simulink model "fil_videosharp_sim"  (R2018b)
settings: Solver=FixedStepDiscrete  StartTime=0.0  StopTime=inf  RelTol=1e-3
InitFcn:
  | filter = fi(fspecial('unsharp'),1,16,12);
  | 
  | % video size excluding the blanking periods
  | fileName = get_param('fil_videosharp_sim/From Multimedia File',  'inputFilename');
  | x=mmfileinfo(fileName);
  | v = x.Video ;
  | H = v.Height;
  | W = v.Width;
  | %H = 176;
  | %W = 240;
  | activeVideoSize = [H W];
  | 
  | % horizontal and vertical blanking
  | hBlanking = 0;
  | vBlanking = 0;
undefined symbols (not defined in the file): gcbh, gray, none, NumBits1, NumBits2, Rec, SDTV, Slope1, Slope2, videoinput
libraries: simulink x19, visionconversions x3, dspsigattribs x3, visiongeotforms x3, dspbuff3 x3, hdlsllib x3, visionsinks x1, dspvision x1, imaqlib x1, simulink_need_slupdate x1, fillib x1
(part 2 of 3)

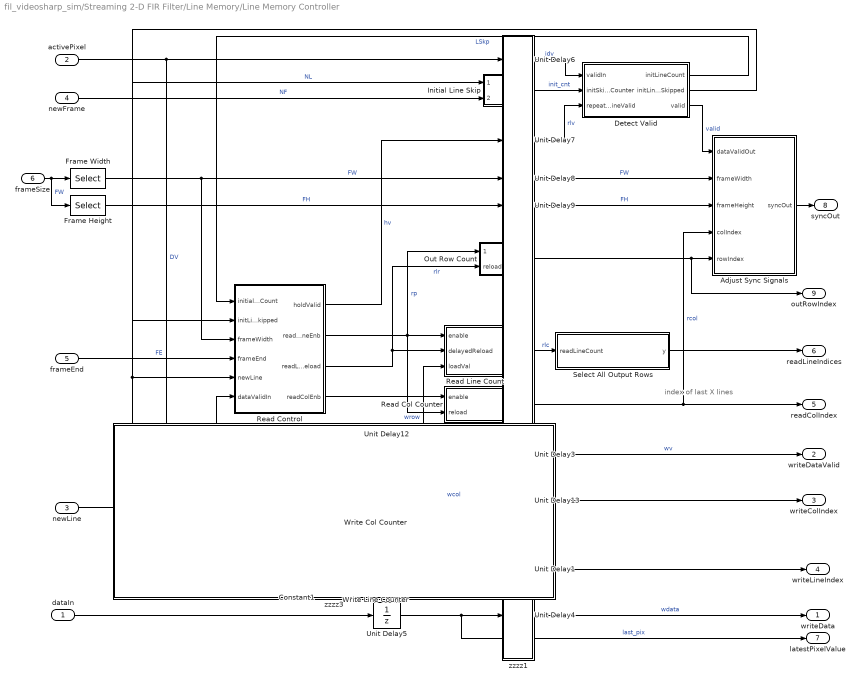
== system fil_videosharp_sim/Streaming 2-D FIR Filter/Line Memory/Line Memory Controller ==
  note: index of last X lines
  dataIn : Inport
  activePixel : Inport  Port=2
  newLine : Inport  Port=3
  newFrame : Inport  Port=4
  frameEnd : Inport  Port=5
  frameSize : Inport  Port=6
  Adjust Sync Signals : Subsystem
  Constant1 : Constant  Value=0  OutDataTypeStr=boolean
  Detect Valid : Subsystem
  Frame Height : Selector  InputPortWidth=2  IndexOptions=Index vector (dialog)  Indices=[1]  OutputSizes=1
  Frame Width : Selector  InputPortWidth=2  IndexOptions=Index vector (dialog)  Indices=[2]  OutputSizes=1
  Initial Line Skip : Subsystem  mask{INIT_VAL=0, STEP_VAL=1, MIN_VAL=0, MAX_VAL=floor(nL/2)+1, RELOADTYPE=Specified reload value, RELOAD_VAL=1, STOPTYPE=stop at specified count, STOP_VAL=floor(nL/2)+1, ROLLTYPE=roll-over to initial value, ROLL_VAL=2, SIGN=unsigned, WLTYPE=auto, WL=10}
      mask prompts: INIT_VAL "Initial value"; STEP_VAL "Step value"; MIN_VAL "Minimum value"; MAX_VAL "Maximum value"; RELOADTYPE "reload to:"; RELOAD_VAL "reload value"; STOPTYPE "Stop at:"; STOP_VAL "Stop at / Roll over from:"; ROLLTYPE "Roll over to:"; ROLL_VAL "Roll-over value"; SIGN "output data is :"; WLTYPE "World length option:"; WL "Word length"
      mask TypeOptions RELOADTYPE: Initial value | Specified reload value
      mask Callback RELOADTYPE:
      | maskStr = get_param(gcb,'MaskValues');
      | maskvisi = get_param(gcb,'MaskVisibilities');
      | maskenebles = get_param(gcb,'MaskEnables');
      | 
      | if strcmp(maskStr{5},'Specified reload value')
      |     maskenebles{6,1}='on';
      |     maskvisi{6,1}='on';
      | else
      |     maskenebles{6,1}='off';
      |     maskvisi{6,1}='off';
      | end
      | 
      | set_param(gcb,'MaskValues',maskStr);
      | set_param(gcb,'MaskVisibilities',maskvisi);
      | set_param(gcb,'MaskEnables',maskenebles);
      mask TypeOptions STOPTYPE: do not stop - auto roll-over | stop at specified count
      mask Callback STOPTYPE:
      | maskStr = get_param(gcb,'MaskValues');
      | maskvisi = get_param(gcb,'MaskVisibilities');
      | maskenebles = get_param(gcb,'MaskEnables');
      | 
      | if strcmp(maskStr{7},'do not stop - auto roll-over')
      |     maskenebles{9,1}='on';
      |     maskvisi{9,1}='on';
      | 
      |     if strcmp(maskStr{9},'roll-over to specified value')
      |         maskenebles{10,1}='on';
      |         maskvisi{10,1}='on';
      |     else
      |         maskenebles{10,1}='off';
      |         maskvisi{10,1}='off';
      | 
      |     end
      | else
      |     maskenebles{9,1}='off';
      |     maskvisi{9,1}='off';
      |     maskenebles{10,1}='off';
      |     maskvisi{10,1}='off';
      | end
      | set_param(gcb,'MaskValues',maskStr);
      | set_param(gcb,'MaskVisibilities',maskvisi);
      | set_param(gcb,'MaskEnables',maskenebles);
      mask TypeOptions ROLLTYPE: roll-over to initial value | roll-over to specified value
      mask Callback ROLLTYPE:
      | maskStr = get_param(gcb,'MaskValues');
      | maskvisi = get_param(gcb,'MaskVisibilities');
      | maskenebles = get_param(gcb,'MaskEnables');
      | 
      | if strcmp(maskStr{9},'roll-over to specified value') ...
      |         && strcmp(maskStr{7},'do not stop - auto roll-over')
      |     maskenebles{10,1}='on';
      |     maskvisi{10,1}='on';
      | else
      |     maskenebles{10,1}='off';
      |     maskvisi{10,1}='off';
      | end
      | 
      | set_param(gcb,'MaskValues',maskStr);
      | set_param(gcb,'MaskVisibilities',maskvisi);
      | set_param(gcb,'MaskEnables',maskenebles);
      mask TypeOptions SIGN: signed | unsigned
      mask TypeOptions WLTYPE: auto | specified
      mask Callback WLTYPE:
      | maskStr = get_param(gcb,'MaskValues');
      | maskvisi = get_param(gcb,'MaskVisibilities');
      | maskenebles = get_param(gcb,'MaskEnables');
      | 
      | if strcmp(maskStr{12},'specified')
      |     maskenebles{13,1}='on';
      |     maskvisi{13,1}='on';
      | else
      |     maskenebles{13,1}='off';
      |     maskvisi{13,1}='off';
      | end
      | 
      | set_param(gcb,'MaskValues',maskStr);
      | set_param(gcb,'MaskVisibilities',maskvisi);
      | set_param(gcb,'MaskEnables',maskenebles);
  Out Row Count : Subsystem  mask{INIT_VAL=0, STEP_VAL=1, MIN_VAL=0, MAX_VAL=maxnr, RELOADTYPE=Initial value, RELOAD_VAL=1, STOPTYPE=stop at specified count, STOP_VAL=maxnr, ROLLTYPE=roll-over to initial value, ROLL_VAL=2, SIGN=unsigned, WLTYPE=auto, WL=10}
      mask prompts: INIT_VAL "Initial value"; STEP_VAL "Step value"; MIN_VAL "Minimum value"; MAX_VAL "Maximum value"; RELOADTYPE "reload to:"; RELOAD_VAL "reload value"; STOPTYPE "Stop at:"; STOP_VAL "Stop at / Roll over from:"; ROLLTYPE "Roll over to:"; ROLL_VAL "Roll-over value"; SIGN "output data is :"; WLTYPE "World length option:"; WL "Word length"
      mask TypeOptions RELOADTYPE: Initial value | Specified reload value
      mask Callback RELOADTYPE:
      | maskStr = get_param(gcb,'MaskValues');
      | maskvisi = get_param(gcb,'MaskVisibilities');
      | maskenebles = get_param(gcb,'MaskEnables');
      | 
      | if strcmp(maskStr{5},'Specified reload value')
      |     maskenebles{6,1}='on';
      |     maskvisi{6,1}='on';
      | else
      |     maskenebles{6,1}='off';
      |     maskvisi{6,1}='off';
      | end
      | 
      | set_param(gcb,'MaskValues',maskStr);
      | set_param(gcb,'MaskVisibilities',maskvisi);
      | set_param(gcb,'MaskEnables',maskenebles);
      mask TypeOptions STOPTYPE: do not stop - auto roll-over | stop at specified count
      mask Callback STOPTYPE:
      | maskStr = get_param(gcb,'MaskValues');
      | maskvisi = get_param(gcb,'MaskVisibilities');
      | maskenebles = get_param(gcb,'MaskEnables');
      | 
      | if strcmp(maskStr{7},'do not stop - auto roll-over')
      |     maskenebles{9,1}='on';
      |     maskvisi{9,1}='on';
      | 
      |     if strcmp(maskStr{9},'roll-over to specified value')
      |         maskenebles{10,1}='on';
      |         maskvisi{10,1}='on';
      |     else
      |         maskenebles{10,1}='off';
      |         maskvisi{10,1}='off';
      | 
      |     end
      | else
      |     maskenebles{9,1}='off';
      |     maskvisi{9,1}='off';
      |     maskenebles{10,1}='off';
      |     maskvisi{10,1}='off';
      | end
      | set_param(gcb,'MaskValues',maskStr);
      | set_param(gcb,'MaskVisibilities',maskvisi);
      | set_param(gcb,'MaskEnables',maskenebles);
      mask TypeOptions ROLLTYPE: roll-over to initial value | roll-over to specified value
      mask Callback ROLLTYPE:
      | maskStr = get_param(gcb,'MaskValues');
      | maskvisi = get_param(gcb,'MaskVisibilities');
      | maskenebles = get_param(gcb,'MaskEnables');
      | 
      | if strcmp(maskStr{9},'roll-over to specified value') ...
      |         && strcmp(maskStr{7},'do not stop - auto roll-over')
      |     maskenebles{10,1}='on';
      |     maskvisi{10,1}='on';
      | else
      |     maskenebles{10,1}='off';
      |     maskvisi{10,1}='off';
      | end
      | 
      | set_param(gcb,'MaskValues',maskStr);
      | set_param(gcb,'MaskVisibilities',maskvisi);
      | set_param(gcb,'MaskEnables',maskenebles);
      mask TypeOptions SIGN: signed | unsigned
      mask TypeOptions WLTYPE: auto | specified
      mask Callback WLTYPE:
      | maskStr = get_param(gcb,'MaskValues');
      | maskvisi = get_param(gcb,'MaskVisibilities');
      | maskenebles = get_param(gcb,'MaskEnables');
      | 
      | if strcmp(maskStr{12},'specified')
      |     maskenebles{13,1}='on';
      |     maskvisi{13,1}='on';
      | else
      |     maskenebles{13,1}='off';
      |     maskvisi{13,1}='off';
      | end
      | 
      | set_param(gcb,'MaskValues',maskStr);
      | set_param(gcb,'MaskVisibilities',maskvisi);
      | set_param(gcb,'MaskEnables',maskenebles);
  Read Col Counter : Subsystem  mask{INIT_VAL=0, STEP_VAL=1, MIN_VAL=0, MAX_VAL=maxnc-1, RELOADTYPE=Initial value, RELOAD_VAL=3, STOPTYPE=stop at specified count, STOP_VAL=maxnc-1, ROLLTYPE=roll-over to specified value, ROLL_VAL=2, SIGN=unsigned, WLTYPE=auto, WL=10}
      mask prompts: INIT_VAL "Initial value"; STEP_VAL "Step value"; MIN_VAL "Minimum value"; MAX_VAL "Maximum value"; RELOADTYPE "reload to:"; RELOAD_VAL "reload value"; STOPTYPE "Stop at:"; STOP_VAL "Stop at / Roll over from:"; ROLLTYPE "Roll over to:"; ROLL_VAL "Roll-over value"; SIGN "output data is :"; WLTYPE "World length option:"; WL "Word length"
      mask TypeOptions RELOADTYPE: Initial value | Specified reload value
      mask Callback RELOADTYPE:
      | maskStr = get_param(gcb,'MaskValues');
      | maskvisi = get_param(gcb,'MaskVisibilities');
      | maskenebles = get_param(gcb,'MaskEnables');
      | 
      | if strcmp(maskStr{5},'Specified reload value')
      |     maskenebles{6,1}='on';
      |     maskvisi{6,1}='on';
      | else
      |     maskenebles{6,1}='off';
      |     maskvisi{6,1}='off';
      | end
      | 
      | set_param(gcb,'MaskValues',maskStr);
      | set_param(gcb,'MaskVisibilities',maskvisi);
      | set_param(gcb,'MaskEnables',maskenebles);
      mask TypeOptions STOPTYPE: do not stop - auto roll-over | stop at specified count
      mask Callback STOPTYPE:
      | maskStr = get_param(gcb,'MaskValues');
      | maskvisi = get_param(gcb,'MaskVisibilities');
      | maskenebles = get_param(gcb,'MaskEnables');
      | 
      | if strcmp(maskStr{7},'do not stop - auto roll-over')
      |     maskenebles{9,1}='on';
      |     maskvisi{9,1}='on';
      | 
      |     if strcmp(maskStr{9},'roll-over to specified value')
      |         maskenebles{10,1}='on';
      |         maskvisi{10,1}='on';
      |     else
      |         maskenebles{10,1}='off';
      |         maskvisi{10,1}='off';
      | 
      |     end
      | else
      |     maskenebles{9,1}='off';
      |     maskvisi{9,1}='off';
      |     maskenebles{10,1}='off';
      |     maskvisi{10,1}='off';
      | end
      | set_param(gcb,'MaskValues',maskStr);
      | set_param(gcb,'MaskVisibilities',maskvisi);
      | set_param(gcb,'MaskEnables',maskenebles);
      mask TypeOptions ROLLTYPE: roll-over to initial value | roll-over to specified value
      mask Callback ROLLTYPE:
      | maskStr = get_param(gcb,'MaskValues');
      | maskvisi = get_param(gcb,'MaskVisibilities');
      | maskenebles = get_param(gcb,'MaskEnables');
      | 
      | if strcmp(maskStr{9},'roll-over to specified value') ...
      |         && strcmp(maskStr{7},'do not stop - auto roll-over')
      |     maskenebles{10,1}='on';
      |     maskvisi{10,1}='on';
      | else
      |     maskenebles{10,1}='off';
      |     maskvisi{10,1}='off';
      | end
      | 
      | set_param(gcb,'MaskValues',maskStr);
      | set_param(gcb,'MaskVisibilities',maskvisi);
      | set_param(gcb,'MaskEnables',maskenebles);
      mask TypeOptions SIGN: signed | unsigned
      mask TypeOptions WLTYPE: auto | specified
      mask Callback WLTYPE:
      | maskStr = get_param(gcb,'MaskValues');
      | maskvisi = get_param(gcb,'MaskVisibilities');
      | maskenebles = get_param(gcb,'MaskEnables');
      | 
      | if strcmp(maskStr{12},'specified')
      |     maskenebles{13,1}='on';
      |     maskvisi{13,1}='on';
      | else
      |     maskenebles{13,1}='off';
      |     maskvisi{13,1}='off';
      | end
      | 
      | set_param(gcb,'MaskValues',maskStr);
      | set_param(gcb,'MaskVisibilities',maskvisi);
      | set_param(gcb,'MaskEnables',maskenebles);
  Read Control : Subsystem
  Read Line Count : Subsystem
  Select All Output Rows : MATLAB Function  TreatAsAtomicUnit=on
  Unit Delay{1,3..9,12..13} (10 alike) : UnitDelay  SampleTime=-1
  Write Col Counter : Subsystem  mask{INIT_VAL=0, STEP_VAL=1, MIN_VAL=0, MAX_VAL=maxnc-1, RELOADTYPE=Initial value, RELOAD_VAL=3, STOPTYPE=stop at specified count, STOP_VAL=maxnc-1, ROLLTYPE=roll-over to specified value, ROLL_VAL=2, SIGN=unsigned, WLTYPE=auto, WL=10}
      mask prompts: INIT_VAL "Initial value"; STEP_VAL "Step value"; MIN_VAL "Minimum value"; MAX_VAL "Maximum value"; RELOADTYPE "reload to:"; RELOAD_VAL "reload value"; STOPTYPE "Stop at:"; STOP_VAL "Stop at / Roll over from:"; ROLLTYPE "Roll over to:"; ROLL_VAL "Roll-over value"; SIGN "output data is :"; WLTYPE "World length option:"; WL "Word length"
      mask TypeOptions RELOADTYPE: Initial value | Specified reload value
      mask Callback RELOADTYPE:
      | maskStr = get_param(gcb,'MaskValues');
      | maskvisi = get_param(gcb,'MaskVisibilities');
      | maskenebles = get_param(gcb,'MaskEnables');
      | 
      | if strcmp(maskStr{5},'Specified reload value')
      |     maskenebles{6,1}='on';
      |     maskvisi{6,1}='on';
      | else
      |     maskenebles{6,1}='off';
      |     maskvisi{6,1}='off';
      | end
      | 
      | set_param(gcb,'MaskValues',maskStr);
      | set_param(gcb,'MaskVisibilities',maskvisi);
      | set_param(gcb,'MaskEnables',maskenebles);
      mask TypeOptions STOPTYPE: do not stop - auto roll-over | stop at specified count
      mask Callback STOPTYPE:
      | maskStr = get_param(gcb,'MaskValues');
      | maskvisi = get_param(gcb,'MaskVisibilities');
      | maskenebles = get_param(gcb,'MaskEnables');
      | 
      | if strcmp(maskStr{7},'do not stop - auto roll-over')
      |     maskenebles{9,1}='on';
      |     maskvisi{9,1}='on';
      | 
      |     if strcmp(maskStr{9},'roll-over to specified value')
      |         maskenebles{10,1}='on';
      |         maskvisi{10,1}='on';
      |     else
      |         maskenebles{10,1}='off';
      |         maskvisi{10,1}='off';
      | 
      |     end
      | else
      |     maskenebles{9,1}='off';
      |     maskvisi{9,1}='off';
      |     maskenebles{10,1}='off';
      |     maskvisi{10,1}='off';
      | end
      | set_param(gcb,'MaskValues',maskStr);
      | set_param(gcb,'MaskVisibilities',maskvisi);
      | set_param(gcb,'MaskEnables',maskenebles);
      mask TypeOptions ROLLTYPE: roll-over to initial value | roll-over to specified value
      mask Callback ROLLTYPE:
      | maskStr = get_param(gcb,'MaskValues');
      | maskvisi = get_param(gcb,'MaskVisibilities');
      | maskenebles = get_param(gcb,'MaskEnables');
      | 
      | if strcmp(maskStr{9},'roll-over to specified value') ...
      |         && strcmp(maskStr{7},'do not stop - auto roll-over')
      |     maskenebles{10,1}='on';
      |     maskvisi{10,1}='on';
      | else
      |     maskenebles{10,1}='off';
      |     maskvisi{10,1}='off';
      | end
      | 
      | set_param(gcb,'MaskValues',maskStr);
      | set_param(gcb,'MaskVisibilities',maskvisi);
      | set_param(gcb,'MaskEnables',maskenebles);
      mask TypeOptions SIGN: signed | unsigned
      mask TypeOptions WLTYPE: auto | specified
      mask Callback WLTYPE:
      | maskStr = get_param(gcb,'MaskValues');
      | maskvisi = get_param(gcb,'MaskVisibilities');
      | maskenebles = get_param(gcb,'MaskEnables');
      | 
      | if strcmp(maskStr{12},'specified')
      |     maskenebles{13,1}='on';
      |     maskvisi{13,1}='on';
      | else
      |     maskenebles{13,1}='off';
      |     maskvisi{13,1}='off';
      | end
      | 
      | set_param(gcb,'MaskValues',maskStr);
      | set_param(gcb,'MaskVisibilities',maskvisi);
      | set_param(gcb,'MaskEnables',maskenebles);
  Write Line Counter : Subsystem  mask{INIT_VAL=0, STEP_VAL=1, MIN_VAL=0, MAX_VAL=nL-1, RELOADTYPE=Initial value, RELOAD_VAL=3, STOPTYPE=do not stop - auto roll-over, STOP_VAL=nL-2, ROLLTYPE=roll-over to initial value, ROLL_VAL=2, SIGN=unsigned, WLTYPE=auto, WL=10}
      mask prompts: INIT_VAL "Initial value"; STEP_VAL "Step value"; MIN_VAL "Minimum value"; MAX_VAL "Maximum value"; RELOADTYPE "reload to:"; RELOAD_VAL "reload value"; STOPTYPE "Stop at:"; STOP_VAL "Stop at / Roll over from:"; ROLLTYPE "Roll over to:"; ROLL_VAL "Roll-over value"; SIGN "output data is :"; WLTYPE "World length option:"; WL "Word length"
      mask TypeOptions RELOADTYPE: Initial value | Specified reload value
      mask Callback RELOADTYPE:
      | maskStr = get_param(gcb,'MaskValues');
      | maskvisi = get_param(gcb,'MaskVisibilities');
      | maskenebles = get_param(gcb,'MaskEnables');
      | 
      | if strcmp(maskStr{5},'Specified reload value')
      |     maskenebles{6,1}='on';
      |     maskvisi{6,1}='on';
      | else
      |     maskenebles{6,1}='off';
      |     maskvisi{6,1}='off';
      | end
      | 
      | set_param(gcb,'MaskValues',maskStr);
      | set_param(gcb,'MaskVisibilities',maskvisi);
      | set_param(gcb,'MaskEnables',maskenebles);
      mask TypeOptions STOPTYPE: do not stop - auto roll-over | stop at specified count
      mask Callback STOPTYPE:
      | maskStr = get_param(gcb,'MaskValues');
      | maskvisi = get_param(gcb,'MaskVisibilities');
      | maskenebles = get_param(gcb,'MaskEnables');
      | 
      | if strcmp(maskStr{7},'do not stop - auto roll-over')
      |     maskenebles{9,1}='on';
      |     maskvisi{9,1}='on';
      | 
      |     if strcmp(maskStr{9},'roll-over to specified value')
      |         maskenebles{10,1}='on';
      |         maskvisi{10,1}='on';
      |     else
      |         maskenebles{10,1}='off';
      |         maskvisi{10,1}='off';
      | 
      |     end
      | else
      |     maskenebles{9,1}='off';
      |     maskvisi{9,1}='off';
      |     maskenebles{10,1}='off';
      |     maskvisi{10,1}='off';
      | end
      | set_param(gcb,'MaskValues',maskStr);
      | set_param(gcb,'MaskVisibilities',maskvisi);
      | set_param(gcb,'MaskEnables',maskenebles);
      mask TypeOptions ROLLTYPE: roll-over to initial value | roll-over to specified value
      mask Callback ROLLTYPE:
      | maskStr = get_param(gcb,'MaskValues');
      | maskvisi = get_param(gcb,'MaskVisibilities');
      | maskenebles = get_param(gcb,'MaskEnables');
      | 
      | if strcmp(maskStr{9},'roll-over to specified value') ...
      |         && strcmp(maskStr{7},'do not stop - auto roll-over')
      |     maskenebles{10,1}='on';
      |     maskvisi{10,1}='on';
      | else
      |     maskenebles{10,1}='off';
      |     maskvisi{10,1}='off';
      | end
      | 
      | set_param(gcb,'MaskValues',maskStr);
      | set_param(gcb,'MaskVisibilities',maskvisi);
      | set_param(gcb,'MaskEnables',maskenebles);
      mask TypeOptions SIGN: signed | unsigned
      mask TypeOptions WLTYPE: auto | specified
      mask Callback WLTYPE:
      | maskStr = get_param(gcb,'MaskValues');
      | maskvisi = get_param(gcb,'MaskVisibilities');
      | maskenebles = get_param(gcb,'MaskEnables');
      | 
      | if strcmp(maskStr{12},'specified')
      |     maskenebles{13,1}='on';
      |     maskvisi{13,1}='on';
      | else
      |     maskenebles{13,1}='off';
      |     maskvisi{13,1}='off';
      | end
      | 
      | set_param(gcb,'MaskValues',maskStr);
      | set_param(gcb,'MaskVisibilities',maskvisi);
      | set_param(gcb,'MaskEnables',maskenebles);
  zzzz1 : Subsystem
      settings: AttributesFormatString=Delay balancing
      mask Display: disp('')
  zzzz3 : Subsystem
      settings: AttributesFormatString=Delay balancing
      mask Display: disp('')
  writeData : Outport
  writeDataValid : Outport  Port=2
  writeColIndex : Outport  Port=3
  writeLineIndex : Outport  Port=4
  readColIndex : Outport  Port=5
  readLineIndices : Outport  Port=6
  latestPixelValue : Outport  Port=7
  syncOut : Outport  Port=8
  outRowIndex : Outport  Port=9
  wires:
  Adjust Sync Signals/1(syncOut) -> syncOut/1
  Unit Delay8/1 -> Adjust Sync Signals/2(frameWidth)  "FW"
  frameSize/1 -> Frame Height/1, Frame Width/1  "FW"
  newFrame/1 -> Initial Line Skip/2(reload)  "NF"
  Detect Valid/2(initLinesSkipped) -> Read Control/2(initLineSkipped)
  Unit Delay1/1 -> writeLineIndex/1
  Unit Delay13/1 -> writeColIndex/1
  Unit Delay12/1 -> Unit Delay3/1
  Read Control/3(readLineReload) -> Out Row Count/2(reload), Read Line Count/2(delayedReload)  "rlr"
  newLine/1 -> Read Control/5(newLine), Initial Line Skip/1(enable), Write Line Counter/1(enable), Write Col Counter/2(reload)  "NL"
  Detect Valid/1(initLineCount) -> Read Control/1(initialLineCount)  "LSkp"
  Unit Delay9/1 -> Adjust Sync Signals/3(frameHeight)  "FH"
  Frame Height/1 -> Unit Delay9/1  "FH"
  Read Control/1(holdValid) -> Unit Delay7/1  "hv"
  frameEnd/1 -> Read Control/4(frameEnd)  "FE"
  Detect Valid/3(valid) -> Adjust Sync Signals/1(dataValidOut)  "valid"
  Unit Delay7/1 -> Detect Valid/3(repeatLineValid)  "rlv"
  Read Control/4(readColEnb) -> Read Col Counter/1(enable)
  Frame Width/1 -> Unit Delay8/1, Read Control/3(frameWidth)  "FW"
  Unit Delay6/1 -> Detect Valid/1(validIn)  "idv"
  Initial Line Skip/1(count) -> Detect Valid/2(initSkipCounter)  "init_cnt"
  Unit Delay4/1 -> writeData/1  "wdata"
  Unit Delay5/1 -> latestPixelValue/1, Unit Delay4/1  "last_pix"
  dataIn/1 -> Unit Delay5/1
  Unit Delay3/1 -> writeDataValid/1  "wv"
  activePixel/1 -> Read Control/6(dataValidIn), Unit Delay12/1, Write Col Counter/1(enable), Unit Delay6/1  "DV"
  Write Col Counter/1(count) -> Unit Delay13/1  "wcol"
  Write Line Counter/1(count) -> Unit Delay1/1, Read Line Count/3(loadVal)  "wrow"
  Read Col Counter/1(count) -> readColIndex/1, Adjust Sync Signals/4(colIndex)  "rcol"
  Select All Output Rows/1(y) -> readLineIndices/1
  Read Line Count/1(count) -> Select All Output Rows/1(readLineCount)  "rlc"
  Constant1/1 -> Write Line Counter/2(reload)
  Out Row Count/1(count) -> Adjust Sync Signals/5(rowIndex), outRowIndex/1
  Read Control/2(readLineEnb) -> Read Col Counter/2(reload), Out Row Count/1(enable), Read Line Count/1(enable)  "rp"

== system fil_videosharp_sim/Streaming 2-D FIR Filter/Line Memory/zzzz3 ==

== system fil_videosharp_sim/Streaming 2-D FIR Filter/Line Memory/zzzz4 ==

== system fil_videosharp_sim/Streaming 2-D FIR Filter/Make Neighborhood/zzzz4 ==

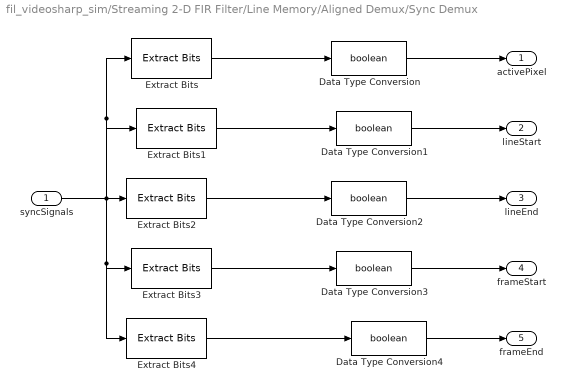
== system fil_videosharp_sim/Streaming 2-D FIR Filter/Line Memory/Aligned Demux/Sync Demux ==
  syncSignals : Inport
  Data Type Conversion{,1..4} (5 alike) : DataTypeConversion  OutDataTypeStr=boolean
  Extract Bits : simulink/Logic and Bit Operations/Extract Bits  bitsToExtract=Range of bits  numBits=8  bitIdxRange=[0]  outScalingMode=Treat bit field as an integer
      settings: SourceProductName=Simulink
  Extract Bits1 : simulink/Logic and Bit Operations/Extract Bits  bitsToExtract=Range of bits  numBits=8  bitIdxRange=[1]  outScalingMode=Treat bit field as an integer
      settings: SourceProductName=Simulink
  Extract Bits2 : simulink/Logic and Bit Operations/Extract Bits  bitsToExtract=Range of bits  numBits=8  bitIdxRange=[2]  outScalingMode=Treat bit field as an integer
      settings: SourceProductName=Simulink
  Extract Bits3 : simulink/Logic and Bit Operations/Extract Bits  bitsToExtract=Range of bits  numBits=8  bitIdxRange=[3]  outScalingMode=Treat bit field as an integer
      settings: SourceProductName=Simulink
  Extract Bits4 : simulink/Logic and Bit Operations/Extract Bits  bitsToExtract=Range of bits  numBits=8  bitIdxRange=[4]  outScalingMode=Treat bit field as an integer
      settings: SourceProductName=Simulink
  activePixel : Outport
  lineStart : Outport  Port=2
  lineEnd : Outport  Port=3
  frameStart : Outport  Port=4
  frameEnd : Outport  Port=5
  wires:
  syncSignals/1 -> Extract Bits/1, Extract Bits1/1, Extract Bits2/1, Extract Bits3/1, Extract Bits4/1
  Extract Bits4/1 -> Data Type Conversion4/1
  Extract Bits3/1 -> Data Type Conversion3/1
  Extract Bits2/1 -> Data Type Conversion2/1
  Extract Bits1/1 -> Data Type Conversion1/1
  Extract Bits/1 -> Data Type Conversion/1
  Data Type Conversion/1 -> activePixel/1
  Data Type Conversion1/1 -> lineStart/1
  Data Type Conversion2/1 -> lineEnd/1
  Data Type Conversion3/1 -> frameStart/1
  Data Type Conversion4/1 -> frameEnd/1

== system fil_videosharp_sim/Streaming 2-D FIR Filter/Line Memory/Line Memory Bank/RAM Blocks  ==
  dataIn : Inport
  writeAdd : Inport  Port=2
  selectWriteRAM : Inport  Port=3
  readAdd : Inport  Port=4
  Dynamic RAM Blocks : Subsystem
      mask init:
      | blk = gcb;  
      | parent = get_param(blk,'parent');
      | %nb = slResolve('nb',parent,'variable');
      | %WL = slResolve('WL',parent,'variable');
      | nb = str2num(get_param(parent,'eval_nb'));
      | WL = str2num(get_param(parent,'eval_WL'));
      | %hws = get_param(bdroot, 'modelworkspace');
      | %nb = hws.evalin('VIPHDL_numb_RAM_block');
      | %WL = hws.evalin('VIPHDL_RAM_block_WL');
      | change_block= true;
      | if change_block
      |       
      |     %find and delete all lines 
      |     blk_paths = find_system(blk,'LookUnderMasks','all','FindAll','on');
      |     if  size(blk_paths,1) >1 
      |       for i=1:size(blk_paths,1) 
      |         if ishandle(blk_paths(i)) 
      |           type = get_param(blk_paths(i),'type');
      |           % fprintf('Id=%d, type=%s\n', i, type);
      |           if ( strcmp(type,'line') )
      |             if ( get_param(blk_paths(i),'LineParent')  == -1 ) 
      |               delete_line(blk_paths(i));
      |             end
      |           end 
      |         end      
      |       end
      |     end
      | 
      |     %find and delete blocks 
      |     blk_paths = find_system(blk,'LookUnderMasks','all','FindAll','off');
      |     if  size(blk_paths,1) >1 
      |       for i=2:size(blk_paths,1)   
      |         type = get_param(blk_paths(i),'type');
      |         if ( strcmp(type,'block') )
      |             blocktype = get_param(blk_paths(i),'BlockType');
      |             if  ~( strcmp(blocktype,'Inport') || strcmp(blocktype,'Outport') )
      |                 blockname = get_param(blk_paths(i),'Name');
      |                 if  ~strcmp(blockname,'RAM1')
      |                   delete_block(blk_paths(i));
      |                 end
      |             end
      |         end
      |       end
      |     end
      | 
      |     % ------- add blocks -------------------
      |     %nram= str2num(get_param(blk,'nb'));
      |     nram= nb ; 
      |     for i= 1:nram
      |       index_sub = num2str(i);
      |       % add selector
      |       name =strcat(blk,'/sel',index_sub); 
      |       location = [125 (100*i) 175 50+(100*i) ];
      |       port_width_str = num2str(nram);
      |       selector_str = strcat('[',num2str(i),']');
      |       add_block('simulink/Signal Routing/Selector',name,'Position',location,'InputPortWidth',... 
      |         port_width_str,'IndexParamArray',{selector_str});
      |       % add data coversion blocks
      |       name =strcat(blk,'/DC',index_sub); 
      |       location = [250 10+(100*i) 300 50-10+(100*i) ];
      |       add_block('simulink/Commonly Used Blocks/Data Type Conversion',name,'Position', ... 
      |         location,'OutDataTypeStr','boolean'); 
      |       % add TAM blocks
      |       name =strcat(blk,'/RAM',index_sub); 
      |       location = [550 -25+(100*i) 650 50+(100*i) ];
      |       src = strcat(blk,'/RAM1');
      |       if (i>1)
      |         add_block(src,name,'Position',location);
      |       end  
      |     end  
      |     % add mux 
      |     name =strcat(blk,'/rMUX'); 
      |     location = [800 230 810 280+(10*nram) ];
      |     add_block('simulink/Signal Routing/Mux',name,'Position',location,'Inputs',num2str(nram));
      | 
      | 
      |     % ------------ add lines ----------------
      |     for i= 1:nram
      |       index_sub = num2str(i);
      |       %selector to DC
      |       src_name =strcat('selectWriteRAM','/1'); 
      |       dest_name =strcat('sel',index_sub,'/1'); 
      |       add_line(blk,src_name,dest_name,'autorouting','on');
      |       %selector to DC
      |       src_name =strcat('sel',index_sub,'/1'); 
      |       dest_name =strcat('DC',index_sub,'/1'); 
      |       add_line(blk,src_name,dest_name,'autorouting','on');
      |       % DC to RAM
      |       src_name =strcat('DC',index_sub,'/1');
      |       dest_name =strcat('RAM',index_sub,'/3');
      |       add_line(blk,src_name,dest_name,'autorouting','on');
      |       % data_in to RAM
      |       src_name =strcat('dataIn','/1');
      |       dest_name =strcat('RAM',index_sub,'/1');
      |       add_line(blk,src_name,dest_name,'autorouting','on');
      |       % write_add to RAM
      |       src_name =strcat('writeAdd','/1');
      |       dest_name =strcat('RAM',index_sub,'/2');
      |       add_line(blk,src_name,dest_name,'autorouting','on');
      |       % read_add to RAM
      |       src_name =strcat('readAdd','/1');
      |       dest_name =strcat('RAM',index_sub,'/4');
      |       add_line(blk,src_name,dest_name,'autorouting','on');
      |       % RAM to Mux
      |       src_name =strcat('RAM',index_sub,'/1');
      |       dest_name =strcat('rMUX/', num2str(i));
      |       add_line(blk,src_name,dest_name,'autorouting','on');  
      |     end
      | 
      |     %mux to output 
      |     src_name ='rMUX/1';
      |     dest_name ='dataOut/1';
      |     add_line(blk,src_name,dest_name,'autorouting','on');   
      | end
  dataOut : Outport
  wires:
  readAdd/1 -> Dynamic RAM Blocks/4(readAdd)
  selectWriteRAM/1 -> Dynamic RAM Blocks/3(selectWriteRAM)
  Dynamic RAM Blocks/1(dataOut) -> dataOut/1
  writeAdd/1 -> Dynamic RAM Blocks/2(writeAdd)
  dataIn/1 -> Dynamic RAM Blocks/1(dataIn)

== system fil_videosharp_sim/Streaming 2-D FIR Filter/Line Memory/Line Memory Bank/zzzz2 ==

== system fil_videosharp_sim/Streaming 2-D FIR Filter/Line Memory/Line Memory Controller/Adjust Sync Signals ==
  dataValidOut : Inport
  frameWidth : Inport  Port=2
  frameHeight : Inport  Port=3
  colIndex : Inport  Port=4
  rowIndex : Inport  Port=5
  Detect Frame End : Subsystem
  Detect Frame Start : Subsystem
  Detect Line End : Subsystem
  Detect Line Start : Subsystem
  SyncMux : Subsystem
  syncOut : Outport
  wires:
  SyncMux/1(syncOut) -> syncOut/1
  Detect Frame Start/1(alignedFrameStart) -> SyncMux/4(FrameStart)
  Detect Frame End/1(valid) -> SyncMux/5(FrameEnd)
  frameHeight/1 -> Detect Frame End/2(frameHeight)
  frameWidth/1 -> Detect Line End/2(frameWidth)
  rowIndex/1 -> Detect Frame Start/2(rowIndex), Detect Frame End/3(rowIndex)
  colIndex/1 -> Detect Line Start/2(colIndex), Detect Line End/3(colIndex)
  dataValidOut/1 -> SyncMux/1(activePixel), Detect Line Start/1(dataValidOut), Detect Line End/1(dataValidOut)
  Detect Line Start/1(alignedLineStart) -> SyncMux/2(lineStart), Detect Frame Start/1(lineStart)
  Detect Line End/1(lineEnd) -> SyncMux/3(lineEnd), Detect Frame End/1(lineEnd)

== system fil_videosharp_sim/Streaming 2-D FIR Filter/Line Memory/Line Memory Controller/Detect Valid ==
  validIn : Inport
  initSkipCounter : Inport  Port=2
  repeatLineValid : Inport  Port=3
  AND : Logic  AllPortsSameDT=off  OutDataTypeStr=boolean
  Compare To Constant1 : simulink/Logic and Bit Operations/Compare To Constant  relop=>  const=floor(nL/2)  OutDataTypeStr=boolean  ZeroCross=off
  OR2 : Logic  Operator=OR  AllPortsSameDT=off  OutDataTypeStr=boolean
  initLineCount : Outport
  initLinesSkipped : Outport  Port=2
  valid : Outport  Port=3
  wires:
  validIn/1 -> AND/2
  AND/1 -> OR2/1
  repeatLineValid/1 -> OR2/2
  OR2/1 -> valid/1
  initSkipCounter/1 -> initLineCount/1, Compare To Constant1/1  "init_count"
  Compare To Constant1/1 -> initLinesSkipped/1, AND/1

== system fil_videosharp_sim/Streaming 2-D FIR Filter/Line Memory/Line Memory Controller/Initial Line Skip ==
  enable : Inport
  reload : Inport  Port=2
  DataTypeConversion : DataTypeConversion  OutDataTypeStr=fixdt(SIGN==1,((WLTYPE==1) * ( ceil(log2(MAX_VAL-MIN_VAL+1)) + double(SIGN==1) ) ) + ((WLTYPE~=1)* WL ),0)
  Unit Delay : UnitDelay  InitialCondition=INIT_VAL  SampleTime=-1
  eML Counter : MATLAB Function  TreatAsAtomicUnit=on
  count : Outport
  wires:
  enable/1 -> eML Counter/2(enb)
  reload/1 -> eML Counter/3(reload)
  Unit Delay/1 -> eML Counter/1(currentCount), count/1
  eML Counter/1(nextCount) -> DataTypeConversion/1
  DataTypeConversion/1 -> Unit Delay/1

== system fil_videosharp_sim/Streaming 2-D FIR Filter/Line Memory/Line Memory Controller/Out Row Count ==
  enable : Inport
  reload : Inport  Port=2
  DataTypeConversion : DataTypeConversion  OutDataTypeStr=fixdt(SIGN==1,((WLTYPE==1) * ( ceil(log2(MAX_VAL-MIN_VAL+1)) + double(SIGN==1) ) ) + ((WLTYPE~=1)* WL ),0)
  Unit Delay : UnitDelay  InitialCondition=INIT_VAL  SampleTime=-1
  eML Counter : MATLAB Function  TreatAsAtomicUnit=on
  count : Outport
  wires:
  DataTypeConversion/1 -> Unit Delay/1
  eML Counter/1(nextCount) -> DataTypeConversion/1
  Unit Delay/1 -> eML Counter/1(currentCount), count/1
  reload/1 -> eML Counter/3(reload)
  enable/1 -> eML Counter/2(enb)

== system fil_videosharp_sim/Streaming 2-D FIR Filter/Line Memory/Line Memory Controller/Read Col Counter ==
  enable : Inport
  reload : Inport  Port=2
  DataTypeConversion : DataTypeConversion  OutDataTypeStr=fixdt(SIGN==1,((WLTYPE==1) * ( ceil(log2(MAX_VAL-MIN_VAL+1)) + double(SIGN==1) ) ) + ((WLTYPE~=1)* WL ),0)
  Unit Delay : UnitDelay  InitialCondition=INIT_VAL  SampleTime=-1
  eML Counter : MATLAB Function  TreatAsAtomicUnit=on
  count : Outport
  wires:
  enable/1 -> eML Counter/2(enb)
  reload/1 -> eML Counter/3(reload)
  Unit Delay/1 -> eML Counter/1(currentCount), count/1
  eML Counter/1(nextCount) -> DataTypeConversion/1
  DataTypeConversion/1 -> Unit Delay/1

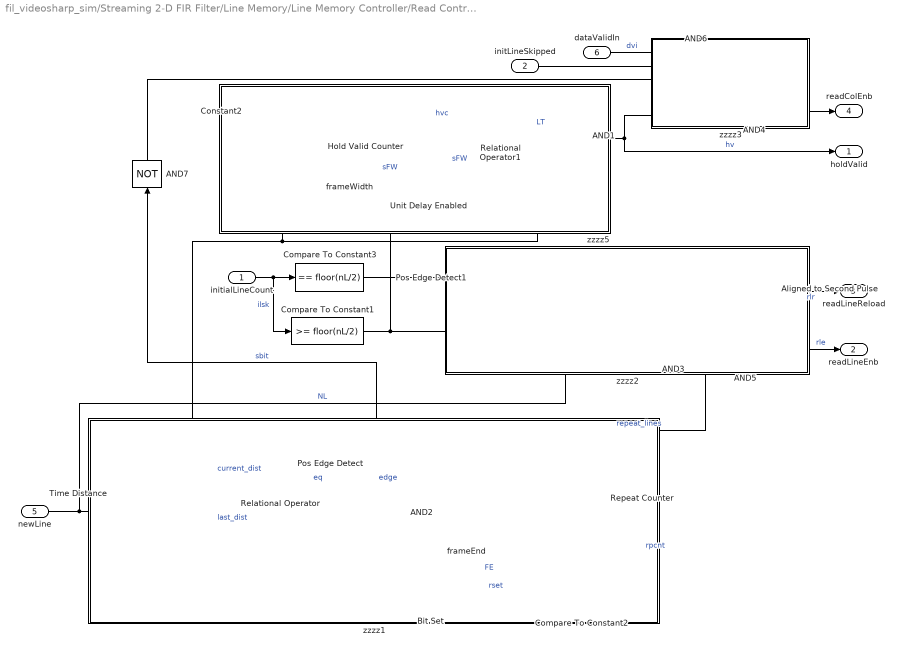
== system fil_videosharp_sim/Streaming 2-D FIR Filter/Line Memory/Line Memory Controller/Read Control ==
  initialLineCount : Inport
  initLineSkipped : Inport  Port=2
  frameWidth : Inport  Port=3
  frameEnd : Inport  Port=4
  newLine : Inport  Port=5
  dataValidIn : Inport  Port=6
  AND1 : Logic  Operator=OR  AllPortsSameDT=off  OutDataTypeStr=boolean
  AND2 : Logic  AllPortsSameDT=off  OutDataTypeStr=boolean
  AND3 : Logic  AllPortsSameDT=off  OutDataTypeStr=boolean
  AND4 : Logic  Operator=OR  AllPortsSameDT=off  OutDataTypeStr=boolean
  AND5 : Logic  Operator=OR  AllPortsSameDT=off  OutDataTypeStr=boolean
  AND6 : Logic  Inputs=3  AllPortsSameDT=off  OutDataTypeStr=boolean
  AND7 : Logic  Operator=NOT  AllPortsSameDT=off  OutDataTypeStr=boolean
  Aligned to Second Pulse : MATLAB Function  TreatAsAtomicUnit=on
  Bit Set : MATLAB Function  TreatAsAtomicUnit=on
  Compare To Constant1 : simulink/Logic and Bit Operations/Compare To Constant  relop=>=  const=floor(nL/2)  OutDataTypeStr=boolean  ZeroCross=off
  Compare To Constant2 : simulink/Logic and Bit Operations/Compare To Constant  relop=>  const=floor(nL/2)-1  OutDataTypeStr=boolean  ZeroCross=off
  Compare To Constant3 : simulink/Logic and Bit Operations/Compare To Constant  relop===  const=floor(nL/2)  OutDataTypeStr=boolean  ZeroCross=off
  Constant2 : Constant  OutDataTypeStr=boolean
  Hold Valid Counter : Subsystem  mask{INIT_VAL=maxnc, STEP_VAL=1, MIN_VAL=0, MAX_VAL=maxnc, RELOADTYPE=Specified reload value, RELOAD_VAL=1, STOPTYPE=stop at specified count, STOP_VAL=maxnc, ROLLTYPE=roll-over to initial value, ROLL_VAL=2, SIGN=unsigned, WLTYPE=auto, WL=10}
      mask prompts: INIT_VAL "Initial value"; STEP_VAL "Step value"; MIN_VAL "Minimum value"; MAX_VAL "Maximum value"; RELOADTYPE "reload to:"; RELOAD_VAL "reload value"; STOPTYPE "Stop at:"; STOP_VAL "Stop at / Roll over from:"; ROLLTYPE "Roll over to:"; ROLL_VAL "Roll-over value"; SIGN "output data is :"; WLTYPE "World length option:"; WL "Word length"
      mask TypeOptions RELOADTYPE: Initial value | Specified reload value
      mask Callback RELOADTYPE:
      | maskStr = get_param(gcb,'MaskValues');
      | maskvisi = get_param(gcb,'MaskVisibilities');
      | maskenebles = get_param(gcb,'MaskEnables');
      | 
      | if strcmp(maskStr{5},'Specified reload value')
      |     maskenebles{6,1}='on';
      |     maskvisi{6,1}='on';
      | else
      |     maskenebles{6,1}='off';
      |     maskvisi{6,1}='off';
      | end
      | 
      | set_param(gcb,'MaskValues',maskStr);
      | set_param(gcb,'MaskVisibilities',maskvisi);
      | set_param(gcb,'MaskEnables',maskenebles);
      mask TypeOptions STOPTYPE: do not stop - auto roll-over | stop at specified count
      mask Callback STOPTYPE:
      | maskStr = get_param(gcb,'MaskValues');
      | maskvisi = get_param(gcb,'MaskVisibilities');
      | maskenebles = get_param(gcb,'MaskEnables');
      | 
      | if strcmp(maskStr{7},'do not stop - auto roll-over')
      |     maskenebles{9,1}='on';
      |     maskvisi{9,1}='on';
      | 
      |     if strcmp(maskStr{9},'roll-over to specified value')
      |         maskenebles{10,1}='on';
      |         maskvisi{10,1}='on';
      |     else
      |         maskenebles{10,1}='off';
      |         maskvisi{10,1}='off';
      | 
      |     end
      | else
      |     maskenebles{9,1}='off';
      |     maskvisi{9,1}='off';
      |     maskenebles{10,1}='off';
      |     maskvisi{10,1}='off';
      | end
      | set_param(gcb,'MaskValues',maskStr);
      | set_param(gcb,'MaskVisibilities',maskvisi);
      | set_param(gcb,'MaskEnables',maskenebles);
      mask TypeOptions ROLLTYPE: roll-over to initial value | roll-over to specified value
      mask Callback ROLLTYPE:
      | maskStr = get_param(gcb,'MaskValues');
      | maskvisi = get_param(gcb,'MaskVisibilities');
      | maskenebles = get_param(gcb,'MaskEnables');
      | 
      | if strcmp(maskStr{9},'roll-over to specified value') ...
      |         && strcmp(maskStr{7},'do not stop - auto roll-over')
      |     maskenebles{10,1}='on';
      |     maskvisi{10,1}='on';
      | else
      |     maskenebles{10,1}='off';
      |     maskvisi{10,1}='off';
      | end
      | 
      | set_param(gcb,'MaskValues',maskStr);
      | set_param(gcb,'MaskVisibilities',maskvisi);
      | set_param(gcb,'MaskEnables',maskenebles);
      mask TypeOptions SIGN: signed | unsigned
      mask TypeOptions WLTYPE: auto | specified
      mask Callback WLTYPE:
      | maskStr = get_param(gcb,'MaskValues');
      | maskvisi = get_param(gcb,'MaskVisibilities');
      | maskenebles = get_param(gcb,'MaskEnables');
      | 
      | if strcmp(maskStr{12},'specified')
      |     maskenebles{13,1}='on';
      |     maskvisi{13,1}='on';
      | else
      |     maskenebles{13,1}='off';
      |     maskvisi{13,1}='off';
      | end
      | 
      | set_param(gcb,'MaskValues',maskStr);
      | set_param(gcb,'MaskVisibilities',maskvisi);
      | set_param(gcb,'MaskEnables',maskenebles);
  Pos Edge Detect : Subsystem
  Pos Edge Detect1 : Subsystem
  Relational Operator : RelationalOperator  Operator===  OutDataTypeStr=boolean  RndMeth=Nearest
  Relational Operator1 : RelationalOperator  Operator=<  OutDataTypeStr=boolean  RndMeth=Nearest
  Repeat Counter : Subsystem  mask{INIT_VAL=0, STEP_VAL=1, MIN_VAL=0, MAX_VAL=floor(nL/2)+1, RELOADTYPE=Specified reload value, RELOAD_VAL=0, STOPTYPE=stop at specified count, STOP_VAL=floor(nL/2)+1, ROLLTYPE=roll-over to initial value, ROLL_VAL=2, SIGN=unsigned, WLTYPE=auto, WL=10}
      mask prompts: INIT_VAL "Initial value"; STEP_VAL "Step value"; MIN_VAL "Minimum value"; MAX_VAL "Maximum value"; RELOADTYPE "reload to:"; RELOAD_VAL "reload value"; STOPTYPE "Stop at:"; STOP_VAL "Stop at / Roll over from:"; ROLLTYPE "Roll over to:"; ROLL_VAL "Roll-over value"; SIGN "output data is :"; WLTYPE "World length option:"; WL "Word length"
      mask TypeOptions RELOADTYPE: Initial value | Specified reload value
      mask Callback RELOADTYPE:
      | maskStr = get_param(gcb,'MaskValues');
      | maskvisi = get_param(gcb,'MaskVisibilities');
      | maskenebles = get_param(gcb,'MaskEnables');
      | 
      | if strcmp(maskStr{5},'Specified reload value')
      |     maskenebles{6,1}='on';
      |     maskvisi{6,1}='on';
      | else
      |     maskenebles{6,1}='off';
      |     maskvisi{6,1}='off';
      | end
      | 
      | set_param(gcb,'MaskValues',maskStr);
      | set_param(gcb,'MaskVisibilities',maskvisi);
      | set_param(gcb,'MaskEnables',maskenebles);
      mask TypeOptions STOPTYPE: do not stop - auto roll-over | stop at specified count
      mask Callback STOPTYPE:
      | maskStr = get_param(gcb,'MaskValues');
      | maskvisi = get_param(gcb,'MaskVisibilities');
      | maskenebles = get_param(gcb,'MaskEnables');
      | 
      | if strcmp(maskStr{7},'do not stop - auto roll-over')
      |     maskenebles{9,1}='on';
      |     maskvisi{9,1}='on';
      | 
      |     if strcmp(maskStr{9},'roll-over to specified value')
      |         maskenebles{10,1}='on';
      |         maskvisi{10,1}='on';
      |     else
      |         maskenebles{10,1}='off';
      |         maskvisi{10,1}='off';
      | 
      |     end
      | else
      |     maskenebles{9,1}='off';
      |     maskvisi{9,1}='off';
      |     maskenebles{10,1}='off';
      |     maskvisi{10,1}='off';
      | end
      | set_param(gcb,'MaskValues',maskStr);
      | set_param(gcb,'MaskVisibilities',maskvisi);
      | set_param(gcb,'MaskEnables',maskenebles);
      mask TypeOptions ROLLTYPE: roll-over to initial value | roll-over to specified value
      mask Callback ROLLTYPE:
      | maskStr = get_param(gcb,'MaskValues');
      | maskvisi = get_param(gcb,'MaskVisibilities');
      | maskenebles = get_param(gcb,'MaskEnables');
      | 
      | if strcmp(maskStr{9},'roll-over to specified value') ...
      |         && strcmp(maskStr{7},'do not stop - auto roll-over')
      |     maskenebles{10,1}='on';
      |     maskvisi{10,1}='on';
      | else
      |     maskenebles{10,1}='off';
      |     maskvisi{10,1}='off';
      | end
      | 
      | set_param(gcb,'MaskValues',maskStr);
      | set_param(gcb,'MaskVisibilities',maskvisi);
      | set_param(gcb,'MaskEnables',maskenebles);
      mask TypeOptions SIGN: signed | unsigned
      mask TypeOptions WLTYPE: auto | specified
      mask Callback WLTYPE:
      | maskStr = get_param(gcb,'MaskValues');
      | maskvisi = get_param(gcb,'MaskVisibilities');
      | maskenebles = get_param(gcb,'MaskEnables');
      | 
      | if strcmp(maskStr{12},'specified')
      |     maskenebles{13,1}='on';
      |     maskvisi{13,1}='on';
      | else
      |     maskenebles{13,1}='off';
      |     maskvisi{13,1}='off';
      | end
      | 
      | set_param(gcb,'MaskValues',maskStr);
      | set_param(gcb,'MaskVisibilities',maskvisi);
      | set_param(gcb,'MaskEnables',maskenebles);
  Time Distance : Subsystem
  Unit Delay Enabled : simulink_need_slupdate/Unit Delay Enabled  vinit=0.0  tsamp=-1
      settings: SourceProductName=Simulink  SourceProductBaseCode=SL
  zzzz1 : Subsystem
      settings: AttributesFormatString=Delay balancing
      mask Display: disp('')
  zzzz2 : Subsystem
      settings: AttributesFormatString=Delay balancing
      mask Display: disp('')
  zzzz3 : Subsystem
      settings: AttributesFormatString=Delay balancing
      mask Display: disp('')
  zzzz5 : Subsystem
      settings: AttributesFormatString=Delay balancing
      mask Display: disp('')
  holdValid : Outport
  readLineEnb : Outport  Port=2
  readLineReload : Outport  Port=3
  readColEnb : Outport  Port=4
  wires:
  initLineSkipped/1 -> AND6/2
  Compare To Constant3/1 -> Pos Edge Detect1/1(x)
  Compare To Constant1/1 -> AND3/1, Unit Delay Enabled/2
  Aligned to Second Pulse/1(out) -> readLineReload/1  "rlr"
  AND7/1 -> AND6/3
  AND6/1 -> AND4/1
  dataValidIn/1 -> AND6/1  "dvi"
  AND4/1 -> readColEnb/1
  Pos Edge Detect1/1(y) -> Aligned to Second Pulse/1(earlyPulse)
  AND5/1 -> readLineEnb/1  "rle"
  AND3/1 -> AND5/1
  initialLineCount/1 -> Compare To Constant3/1, Compare To Constant1/1  "ilsk"
  Unit Delay Enabled/1 -> Relational Operator1/2  "sFW"
  AND1/1 -> holdValid/1, AND4/2  "hv"
  Compare To Constant2/1 -> Bit Set/2(reset)  "rset"
  Repeat Counter/1(count) -> Compare To Constant2/1  "rpcnt"
  frameEnd/1 -> Bit Set/1(set), Repeat Counter/2(reload)  "FE"
  AND2/1 -> Repeat Counter/1(enable), AND1/2, Hold Valid Counter/2(reload), Time Distance/1(repeat), AND5/2  "repeat_lines"
  Relational Operator1/1 -> AND1/1  "LT"
  frameWidth/1 -> Unit Delay Enabled/1  "sFW"
  newLine/1 -> Aligned to Second Pulse/2(latePulse), AND3/2, Time Distance/2(newLine)  "NL"
  Hold Valid Counter/1(count) -> Relational Operator1/1  "hvc"
  Constant2/1 -> Hold Valid Counter/1(enable)
  Time Distance/2(lastDistance) -> Relational Operator/2  "last_dist"
  Time Distance/1(currentDistance) -> Relational Operator/1  "current_dist"
  Pos Edge Detect/1(y) -> AND2/1  "edge"
  Relational Operator/1 -> Pos Edge Detect/1(x)  "eq"
  Bit Set/1(status) -> AND2/2, AND7/1  "sbit"

== system fil_videosharp_sim/Streaming 2-D FIR Filter/Line Memory/Line Memory Controller/Read Line Count ==
  enable : Inport
  delayedReload : Inport  Port=2
  loadVal : Inport  Port=3
  Multiport Switch : MultiPortSwitch  DataPortOrder=Zero-based contiguous  Inputs=2  zeroidx=on
  Read Line Counter1 : Subsystem  mask{INIT_VAL=0, STEP_VAL=1, MIN_VAL=0, MAX_VAL=nL-1, RELOADTYPE=Initial value, RELOAD_VAL=3, STOPTYPE=do not stop - auto roll-over, STOP_VAL=nL-2, ROLLTYPE=roll-over to initial value, ROLL_VAL=2, SIGN=unsigned, WLTYPE=auto, WL=10}
      mask prompts: INIT_VAL "Initial value"; STEP_VAL "Step value"; MIN_VAL "Minimum value"; MAX_VAL "Maximum value"; RELOADTYPE "reload to:"; RELOAD_VAL "reload value"; STOPTYPE "Stop at:"; STOP_VAL "Stop at / Roll over from:"; ROLLTYPE "Roll over to:"; ROLL_VAL "Roll-over value"; SIGN "output data is :"; WLTYPE "World length option:"; WL "Word length"
      mask TypeOptions RELOADTYPE: Initial value | Specified reload value
      mask Callback RELOADTYPE:
      | maskStr = get_param(gcb,'MaskValues');
      | maskvisi = get_param(gcb,'MaskVisibilities');
      | maskenebles = get_param(gcb,'MaskEnables');
      | 
      | if strcmp(maskStr{5},'Specified reload value')
      |     maskenebles{6,1}='on';
      |     maskvisi{6,1}='on';
      | else
      |     maskenebles{6,1}='off';
      |     maskvisi{6,1}='off';
      | end
      | 
      | set_param(gcb,'MaskValues',maskStr);
      | set_param(gcb,'MaskVisibilities',maskvisi);
      | set_param(gcb,'MaskEnables',maskenebles);
      mask TypeOptions STOPTYPE: do not stop - auto roll-over | stop at specified count
      mask Callback STOPTYPE:
      | maskStr = get_param(gcb,'MaskValues');
      | maskvisi = get_param(gcb,'MaskVisibilities');
      | maskenebles = get_param(gcb,'MaskEnables');
      | 
      | if strcmp(maskStr{7},'do not stop - auto roll-over')
      |     maskenebles{9,1}='on';
      |     maskvisi{9,1}='on';
      | 
      |     if strcmp(maskStr{9},'roll-over to specified value')
      |         maskenebles{10,1}='on';
      |         maskvisi{10,1}='on';
      |     else
      |         maskenebles{10,1}='off';
      |         maskvisi{10,1}='off';
      | 
      |     end
      | else
      |     maskenebles{9,1}='off';
      |     maskvisi{9,1}='off';
      |     maskenebles{10,1}='off';
      |     maskvisi{10,1}='off';
      | end
      | set_param(gcb,'MaskValues',maskStr);
      | set_param(gcb,'MaskVisibilities',maskvisi);
      | set_param(gcb,'MaskEnables',maskenebles);
      mask TypeOptions ROLLTYPE: roll-over to initial value | roll-over to specified value
      mask Callback ROLLTYPE:
      | maskStr = get_param(gcb,'MaskValues');
      | maskvisi = get_param(gcb,'MaskVisibilities');
      | maskenebles = get_param(gcb,'MaskEnables');
      | 
      | if strcmp(maskStr{9},'roll-over to specified value') ...
      |         && strcmp(maskStr{7},'do not stop - auto roll-over')
      |     maskenebles{10,1}='on';
      |     maskvisi{10,1}='on';
      | else
      |     maskenebles{10,1}='off';
      |     maskvisi{10,1}='off';
      | end
      | 
      | set_param(gcb,'MaskValues',maskStr);
      | set_param(gcb,'MaskVisibilities',maskvisi);
      | set_param(gcb,'MaskEnables',maskenebles);
      mask TypeOptions SIGN: signed | unsigned
      mask TypeOptions WLTYPE: auto | specified
      mask Callback WLTYPE:
      | maskStr = get_param(gcb,'MaskValues');
      | maskvisi = get_param(gcb,'MaskVisibilities');
      | maskenebles = get_param(gcb,'MaskEnables');
      | 
      | if strcmp(maskStr{12},'specified')
      |     maskenebles{13,1}='on';
      |     maskvisi{13,1}='on';
      | else
      |     maskenebles{13,1}='off';
      |     maskvisi{13,1}='off';
      | end
      | 
      | set_param(gcb,'MaskValues',maskStr);
      | set_param(gcb,'MaskVisibilities',maskvisi);
      | set_param(gcb,'MaskEnables',maskenebles);
  Unit Delay8 : UnitDelay  SampleTime=-1
  count : Outport
  wires:
  Multiport Switch/1 -> count/1
  Read Line Counter1/1(count) -> Multiport Switch/2
  Unit Delay8/1 -> Multiport Switch/1, Read Line Counter1/2(reload)
  loadVal/1 -> Multiport Switch/3, Read Line Counter1/3(loadVal)
  delayedReload/1 -> Unit Delay8/1
  enable/1 -> Read Line Counter1/1(enable)
